simulink model "gm_uz_mpc_cost_and_optim_state_machine"  (R2021a)
settings: Solver=FixedStepAuto  StartTime=0.0  StopTime=10000*t_ADC  RelTol=1e-3
undefined symbols (not defined in the file or in its folder): A, f, IB, id_ref, iq_ref, ix_ref, iy_ref, lambda_d, lambda_q, lambda_u, lambda_x, lambda_y, Ld_over_LB, Lq_over_LB, n_rpm, omega_m, omegaB, p, psi_pm_over_psiB, Rs_over_ZB, t_ADC, t_clock, Ts_times_ZB_over_Ld, Ts_times_ZB_over_Lq, Ts_times_ZB_over_Lx, Ts_times_ZB_over_Ly, v_dc, VB
libraries: hdlmdlgenlib x73, nesl_utility x38, fl_lib x30, ee_lib x14, simulink x10, hdlsllib x2
(part 2 of 3)

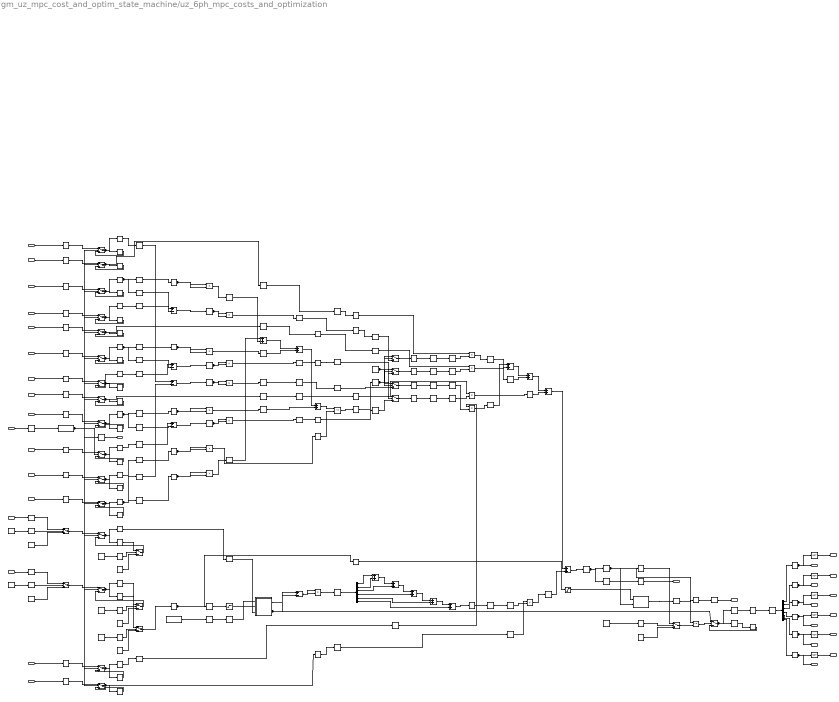
== system gm_uz_mpc_cost_and_optim_state_machine/uz_6ph_mpc_costs_and_optimization ==
  note: squared current error
  note: check for current limit violation
  note: calculate switching effort
  note: calculate costs
  note: find minimum of costs by comparing costs one after another
  note: i_max^2 <= id^2+iq^2+ix^2+iy^2
  id_ref_pu_AXI : Inport  OutDataTypeStr=fixdt(1, 18, 11)  PortDimensions=1  SampleTime=1e-08
  iq_ref_pu_AXI : Inport  Port=2  OutDataTypeStr=fixdt(1, 18, 11)  PortDimensions=1  SampleTime=1e-08
  ix_ref_pu_AXI : Inport  Port=3  OutDataTypeStr=fixdt(1, 18, 11)  PortDimensions=1  SampleTime=1e-08
  iy_ref_pu_AXI : Inport  Port=4  OutDataTypeStr=fixdt(1, 18, 11)  PortDimensions=1  SampleTime=1e-08
  id_pred_pu : Inport  Port=5  OutDataTypeStr=fixdt(1, 27, 16)  PortDimensions=1  SampleTime=1e-08
  iq_pred_pu : Inport  Port=6  OutDataTypeStr=fixdt(1, 27, 16)  PortDimensions=1  SampleTime=1e-08
  ix_pred_pu : Inport  Port=7  OutDataTypeStr=fixdt(1, 18, 11)  PortDimensions=1  SampleTime=1e-08
  iy_pred_pu : Inport  Port=8  OutDataTypeStr=fixdt(1, 18, 11)  PortDimensions=1  SampleTime=1e-08
  max_current_pu_AXI : Inport  Port=9  OutDataTypeStr=fixdt(0, 18, 15)  PortDimensions=1  SampleTime=1e-08
  index : Inport  Port=10  OutDataTypeStr=uint8  PortDimensions=1  SampleTime=1e-08
  last_optim_index : Inport  Port=11  OutDataTypeStr=uint32  PortDimensions=1  SampleTime=1e-08
  lambda_d_AXI : Inport  Port=12  OutDataTypeStr=fixdt(0, 18, 17)  PortDimensions=1  SampleTime=1e-08
  lambda_q_AXI : Inport  Port=13  OutDataTypeStr=fixdt(0, 18, 17)  PortDimensions=1  SampleTime=1e-08
  lambda_x_AXI : Inport  Port=14  OutDataTypeStr=fixdt(0, 18, 17)  PortDimensions=1  SampleTime=1e-08
  lambda_y_AXI : Inport  Port=15  OutDataTypeStr=fixdt(0, 18, 17)  PortDimensions=1  SampleTime=1e-08
  lambda_u_AXI : Inport  Port=16  OutDataTypeStr=fixdt(0, 18, 17)  PortDimensions=1  SampleTime=1e-08
  trigger : Inport  Port=17  OutDataTypeStr=boolean  PortDimensions=1  SampleTime=1e-08
  Add : Sum  Inputs=+-  AccumDataTypeStr=fixdt(1, 28, 16)  OutDataTypeStr=fixdt(1, 28, 16)  SampleTime=1e-08
  Add1 : Sum  Inputs=+-  AccumDataTypeStr=fixdt(1, 28, 16)  OutDataTypeStr=fixdt(1, 28, 16)  SampleTime=1e-08
  Add2 : Sum  Inputs=+-  AccumDataTypeStr=fixdt(1, 19, 11)  OutDataTypeStr=fixdt(1, 19, 11)  SampleTime=1e-08
  Add3 : Sum  Inputs=+-  AccumDataTypeStr=fixdt(1, 19, 11)  OutDataTypeStr=fixdt(1, 19, 11)  SampleTime=1e-08
  Add4_stage2 : Sum  AccumDataTypeStr=fixdt(0, 27, 22)  OutDataTypeStr=fixdt(0, 28, 22)  SampleTime=1e-08
  Add4_stage3 : Sum  AccumDataTypeStr=fixdt(0, 27, 22)  OutDataTypeStr=fixdt(0, 29, 22)  SampleTime=1e-08
  Add4_stage4 : Sum  AccumDataTypeStr=fixdt(0, 27, 22)  OutDataTypeStr=fixdt(0, 27, 22)  SampleTime=1e-08
  Add5 : Sum  Inputs=+-  AccumDataTypeStr=fixdt(1, 9, 0)  OutDataTypeStr=fixdt(1, 9, 0)  SampleTime=1e-08
  Add6_stage2 : Sum  AccumDataTypeStr=fixdt(0, 27, 24)  OutDataTypeStr=fixdt(0, 28, 22)  SampleTime=1e-08
  Add6_stage3 : Sum  AccumDataTypeStr=fixdt(0, 27, 24)  OutDataTypeStr=fixdt(0, 29, 22)  SampleTime=1e-08
  Add6_stage4 : Sum  AccumDataTypeStr=fixdt(0, 27, 24)  OutDataTypeStr=fixdt(0, 30, 22)  SampleTime=1e-08
  Add6_stage5 : Sum  AccumDataTypeStr=fixdt(0, 27, 24)  OutDataTypeStr=fixdt(0, 27, 24)  SampleTime=1e-08
  Delay{,1..23,25..49,51..72,94} (72 alike) : Delay  DelayLength=double(1)  InitialCondition=0  SampleTime=1e-08
  Delay13_Initial_Val : Constant  OutDataTypeStr=uint32  SampleTime=1e-08
  Delay13_ctrl_const : Constant  OutDataTypeStr=boolean  SampleTime=1e-08
  Delay13_ctrl_delay : Delay  DelayLength=double(1)  InitialCondition=0  SampleTime=1e-08
  Delay13_switch : Switch  Criteria=u2 ~= 0  Threshold=double(0)  OutDataTypeStr=uint32  SampleTime=1e-08
  Delay22_Initial_Val : Constant  OutDataTypeStr=uint32  SampleTime=1e-08
  Delay22_ctrl_const : Constant  OutDataTypeStr=boolean  SampleTime=1e-08
  Delay22_ctrl_delay : Delay  DelayLength=double(1)  InitialCondition=0  SampleTime=1e-08
  Delay22_switch : Switch  Criteria=u2 ~= 0  Threshold=double(0)  OutDataTypeStr=uint32  SampleTime=1e-08
  Delay23_Initial_Val : Constant  OutDataTypeStr=uint8  SampleTime=1e-08
  Delay23_ctrl_const : Constant  OutDataTypeStr=boolean  SampleTime=1e-08
  Delay23_ctrl_delay : Delay  DelayLength=double(1)  InitialCondition=0  SampleTime=1e-08
  Delay23_switch : Switch  Criteria=u2 ~= 0  Threshold=double(0)  OutDataTypeStr=uint8  SampleTime=1e-08
  Delay24 : Delay  DelayLength=double(2)  InitialCondition=0  SampleTime=1e-08
  Delay24_Initial_Val : Constant  OutDataTypeStr=uint8  SampleTime=1e-08
  Delay24_ctrl_const : Constant  OutDataTypeStr=boolean  SampleTime=1e-08
  Delay24_ctrl_delay : Delay  DelayLength=double(2)  InitialCondition=0  SampleTime=1e-08
  Delay24_switch : Switch  Criteria=u2 ~= 0  Threshold=double(0)  OutDataTypeStr=uint8  SampleTime=1e-08
  Delay35_Initial_Val : Constant  Value=4.9900000095367431640625  OutDataTypeStr=fixdt(0, 27, 24)  SampleTime=1e-08
  Delay35_ctrl_const : Constant  OutDataTypeStr=boolean  SampleTime=1e-08
  Delay35_ctrl_delay : Delay  DelayLength=double(1)  InitialCondition=0  SampleTime=1e-08
  Delay35_switch : Switch  Criteria=u2 ~= 0  Threshold=double(0)  OutDataTypeStr=fixdt(0, 27, 24)  SampleTime=1e-08
  Delay37_out1_wire : hdlmdlgenlib/Buffer
      settings: SourceProductBaseCode=SL
  Delay38_out1_0_wire : hdlmdlgenlib/Buffer
      settings: SourceProductBaseCode=SL
  Delay38_out1_1_wire : hdlmdlgenlib/Buffer
      settings: SourceProductBaseCode=SL
  Delay38_out1_2_wire : hdlmdlgenlib/Buffer
      settings: SourceProductBaseCode=SL
  Delay38_out1_3_wire : hdlmdlgenlib/Buffer
      settings: SourceProductBaseCode=SL
  Delay38_out1_4_wire : hdlmdlgenlib/Buffer
      settings: SourceProductBaseCode=SL
  Delay38_out1_5_wire : hdlmdlgenlib/Buffer
      settings: SourceProductBaseCode=SL
  Delay50 : Delay  DelayLength=double(4)  InitialCondition=0  SampleTime=1e-08
  Delay50_Initial_Val : Constant  OutDataTypeStr=uint8  SampleTime=1e-08
  Delay50_ctrl_const : Constant  OutDataTypeStr=boolean  SampleTime=1e-08
  Delay50_ctrl_delay : Delay  DelayLength=double(4)  InitialCondition=0  SampleTime=1e-08
  Delay50_switch : Switch  Criteria=u2 ~= 0  Threshold=double(0)  OutDataTypeStr=uint8  SampleTime=1e-08
  Detect Rise Positive : simulink/Logic and Bit Operations/Detect Rise Positive  vinit=0  OutDataTypeStr=boolean
  FiniteControlSetSwitchingTable : Subsystem
  From{,1..34,36} (36 alike) : hdlmdlgenlib/Buffer
      settings: SourceProductBaseCode=SL
  Goto{,1..27,29,47} (30 alike) : hdlmdlgenlib/Buffer
      settings: SourceProductBaseCode=SL
  MATLAB Function : Subsystem
  NOT{,1..5} (6 alike) : Logic  Operator=NOT  Inputs=1  AllPortsSameDT=off  OutDataTypeStr=boolean  SampleTime=1e-08
  Product{,1..7,9..12,14} (13 alike) : Product  Inputs=**  OutDataTypeStr=fixdt(0, 27, 22)  SampleTime=1e-08
  Product13 : Product  Inputs=**  OutDataTypeStr=fixdt(0, 27, 24)  SampleTime=1e-08
  Product8 : Product  Inputs=**  OutDataTypeStr=uint16  SampleTime=1e-08
  Relational Operator : RelationalOperator  OutDataTypeStr=boolean  SampleTime=1e-08  RndMeth=Nearest
  Relational Operator1 : RelationalOperator  Operator=<=  OutDataTypeStr=boolean  SampleTime=1e-08  RndMeth=Nearest
  Saturation : Saturate  UpperLimit="fi(0,0,8,0,\"hex\",\"40\")"  LowerLimit="fi(0,0,8,0,\"hex\",\"01\")"  SampleTime=1e-08  OutDataTypeStr=uint8
  Saturation1 : Saturate  UpperLimit="fi(0,0,8,0,\"hex\",\"40\")"  LowerLimit="fi(0,0,8,0,\"hex\",\"01\")"  SampleTime=1e-08  OutDataTypeStr=uint8
  Sum of Elements_stage2 : Sum  AccumDataTypeStr=uint16  OutDataTypeStr=fixdt(0, 17, 0)  SampleTime=1e-08
  Sum of Elements_stage3 : Sum  AccumDataTypeStr=uint16  OutDataTypeStr=fixdt(0, 18, 0)  SampleTime=1e-08
  Sum of Elements_stage4 : Sum  AccumDataTypeStr=uint16  OutDataTypeStr=fixdt(0, 19, 0)  SampleTime=1e-08
  Sum of Elements_stage5 : Sum  AccumDataTypeStr=uint16  OutDataTypeStr=fixdt(0, 20, 0)  SampleTime=1e-08
  Sum of Elements_stage6 : Sum  AccumDataTypeStr=uint16  OutDataTypeStr=uint16  SampleTime=1e-08
  Switch{,12..14} (4 alike) : Switch  Criteria=u2 > Threshold  Threshold=double(0)  OutDataTypeStr=fixdt(0, 27, 22)  SampleTime=1e-08
  Switch1 : Switch  Criteria=u2 > Threshold  Threshold=double(0)  OutDataTypeStr=fixdt(1, 27, 16)  SampleTime=1e-08
  Switch10 : Switch  Criteria=u2 > Threshold  Threshold=double(0)  OutDataTypeStr=uint32  SampleTime=1e-08
  Switch11 : Switch  Criteria=u2 > Threshold  Threshold=double(0)  OutDataTypeStr=uint8  SampleTime=1e-08
  Switch{15..19} (5 alike) : Switch  Criteria=u2 > Threshold  Threshold=double(0)  OutDataTypeStr=fixdt(0, 18, 17)  SampleTime=1e-08
  Switch2 : Switch  Criteria=u2 > Threshold  Threshold=double(0)  OutDataTypeStr=fixdt(1, 27, 16)  SampleTime=1e-08
  Switch21 : Switch  Criteria=u2 > Threshold  Threshold=double(0)  OutDataTypeStr=boolean  SampleTime=1e-08
  Switch{3..4,6..9} (6 alike) : Switch  Criteria=u2 > Threshold  Threshold=double(0)  OutDataTypeStr=fixdt(1, 18, 11)  SampleTime=1e-08
  Switch5 : Switch  Criteria=u2 > Threshold  Threshold=double(0)  OutDataTypeStr=fixdt(0, 18, 15)  SampleTime=1e-08
  iterativesearch : Subsystem
  sfix18_En15 max value : Constant  Value=3.989990234375  OutDataTypeStr=fixdt(1, 18, 15)  SampleTime=1e-08
  t : Demux  Outputs=6
  t1 : Demux  Outputs=6
  opt_index : Outport  SampleTime=1e-08  VectorParamsAs1DForOutWhenUnconnected=off
  G0 : Outport  Port=2  SampleTime=1e-08  VectorParamsAs1DForOutWhenUnconnected=off
  G1 : Outport  Port=3  SampleTime=1e-08  VectorParamsAs1DForOutWhenUnconnected=off
  G2 : Outport  Port=4  SampleTime=1e-08  VectorParamsAs1DForOutWhenUnconnected=off
  G3 : Outport  Port=5  SampleTime=1e-08  VectorParamsAs1DForOutWhenUnconnected=off
  G4 : Outport  Port=6  SampleTime=1e-08  VectorParamsAs1DForOutWhenUnconnected=off
  G5 : Outport  Port=7  SampleTime=1e-08  VectorParamsAs1DForOutWhenUnconnected=off
  G6 : Outport  Port=8  SampleTime=1e-08  VectorParamsAs1DForOutWhenUnconnected=off
  G7 : Outport  Port=9  SampleTime=1e-08  VectorParamsAs1DForOutWhenUnconnected=off
  G8 : Outport  Port=10  SampleTime=1e-08  VectorParamsAs1DForOutWhenUnconnected=off
  G9 : Outport  Port=11  SampleTime=1e-08  VectorParamsAs1DForOutWhenUnconnected=off
  G10 : Outport  Port=12  SampleTime=1e-08  VectorParamsAs1DForOutWhenUnconnected=off
  G11 : Outport  Port=13  SampleTime=1e-08  VectorParamsAs1DForOutWhenUnconnected=off
  opt_done : Outport  Port=14  SampleTime=1e-08  VectorParamsAs1DForOutWhenUnconnected=off
  costs : Outport  Port=15  SampleTime=1e-08  VectorParamsAs1DForOutWhenUnconnected=off
  wires:
  id_ref_pu_AXI/1 -> Delay14/1
  iq_ref_pu_AXI/1 -> Delay16/1
  ix_ref_pu_AXI/1 -> Delay18/1
  iy_ref_pu_AXI/1 -> Delay20/1
  id_pred_pu/1 -> Delay2/1
  iq_pred_pu/1 -> Delay5/1
  ix_pred_pu/1 -> Delay7/1
  iy_pred_pu/1 -> Delay9/1
  max_current_pu_AXI/1 -> Delay12/1
  index/1 -> Delay24/1
  last_optim_index/1 -> Delay22/1
  lambda_d_AXI/1 -> Delay26/1
  lambda_q_AXI/1 -> Delay28/1
  lambda_x_AXI/1 -> Delay30/1
  lambda_y_AXI/1 -> Delay32/1
  lambda_u_AXI/1 -> Delay34/1
  trigger/1 -> Delay/1
  Add/1 -> Delay46/1
  Add1/1 -> Delay47/1
  Add2/1 -> Delay48/1
  Add3/1 -> Delay49/1
  Add4_stage4/1 -> Relational Operator/1
  Add5/1 -> Product8/2, Product8/1
  Add6_stage5/1 -> Goto27/1
  Delay/1 -> Detect Rise Positive/1
  Delay1/1 -> opt_done/1
  Delay10/1 -> Switch4/3
  Delay11/1 -> Switch5/3
  Delay12/1 -> Switch5/1
  Delay13_switch/1 -> Switch10/3
  Delay14/1 -> Switch6/1
  Delay15/1 -> Switch6/3
  Delay16/1 -> Switch7/1
  Delay17/1 -> Switch7/3
  Delay18/1 -> Switch8/1
  Delay19/1 -> Switch8/3
  Delay2/1 -> Switch1/1
  Delay20/1 -> Switch9/1
  Delay21/1 -> Switch9/3
  Delay22_switch/1 -> Switch10/1
  Delay23_switch/1 -> Switch11/3
  Delay24_switch/1 -> Switch11/1
  Delay25/1 -> Switch15/3
  Delay26/1 -> Switch15/1
  Delay27/1 -> Switch16/3
  Delay28/1 -> Switch16/1
  Delay29/1 -> Switch17/3
  Delay3/1 -> Switch1/3
  Delay30/1 -> Switch17/1
  Delay31/1 -> Switch18/3
  Delay32/1 -> Switch18/1
  Delay33/1 -> Switch19/3
  Delay34/1 -> Switch19/1
  Delay35_switch/1 -> Relational Operator1/2
  Delay36/1 -> Product4/2, Product4/1
  Delay37/1 -> Delay37_out1_wire/1
  Delay38/1 -> t/1
  Delay39/1 -> Product5/2, Product5/1
  Delay4/1 -> opt_index/1
  Delay40/1 -> Product6/2, Product6/1
  Delay41/1 -> Product7/2, Product7/1
  Delay42/1 -> Add4_stage2/1
  Delay43/1 -> Add4_stage2/2
  Delay44/1 -> Add4_stage3/2
  Delay45/1 -> Add4_stage4/2
  Delay46/1 -> Product/2, Product/1
  Delay47/1 -> Product1/2, Product1/1
  Delay48/1 -> Product2/2, Product2/1
  Delay49/1 -> Product3/2, Product3/1
  Delay5/1 -> Switch2/1
  Delay50_switch/1 -> Goto2/1
  Delay51/1 -> Product14/2, Product14/1
  Delay52/1 -> Relational Operator/2
  Delay53/1 -> Add6_stage2/1
  Delay54/1 -> Add6_stage2/2
  Delay55/1 -> Add6_stage3/2
  Delay56/1 -> Add6_stage4/2
  Delay57/1 -> Add6_stage5/2
  Delay58/1 -> t1/1
  Delay59/1 -> Product9/2
  Delay6/1 -> Switch2/3
  Delay60/1 -> Product10/2
  Delay61/1 -> Product11/2
  Delay62/1 -> Product12/2
  Delay63/1 -> Product13/2
  Delay64/1 -> Product9/1
  Delay65/1 -> Product10/1
  Delay66/1 -> Product11/1
  Delay67/1 -> Product12/1
  Delay68/1 -> Product13/1
  Delay69/1 -> Goto10/1
  Delay7/1 -> Switch3/1
  Delay70/1 -> Goto11/1
  Delay71/1 -> Goto12/1
  Delay72/1 -> Goto13/1
  Delay8/1 -> Switch3/3
  Delay9/1 -> Switch4/1
  Delay94/1 -> costs/1
  Delay38_out1_0_wire/1 -> NOT/1, G0/1
  Delay38_out1_1_wire/1 -> NOT1/1, G2/1
  Delay38_out1_2_wire/1 -> NOT2/1, G4/1
  Delay38_out1_3_wire/1 -> NOT3/1, G6/1
  Delay38_out1_4_wire/1 -> NOT4/1, G8/1
  Delay38_out1_5_wire/1 -> NOT5/1, G10/1
  Detect Rise Positive/1 -> Switch9/2, Switch8/2, Switch7/2, Switch6/2, Switch5/2, Switch4/2, Switch3/2, Switch2/2, Switch19/2, Switch18/2, Switch17/2, Switch16/2, Switch15/2, Switch11/2, Switch10/2, Switch1/2, Delay1/1
  FiniteControlSetSwitchingTable/1(G) -> Goto47/1
  From/1 -> Add/1
  From1/1 -> Add/2
  From10/1 -> Switch/3
  From11/1 -> Switch14/2, Switch13/2, Switch12/2, Switch/2
  From12/1 -> Switch12/3
  From13/1 -> Switch13/3
  From14/1 -> Delay36/1
  From15/1 -> Delay39/1
  From16/1 -> Delay40/1
  From17/1 -> Delay41/1
  From18/1 -> Switch14/3
  From19/1 -> Saturation/1
  From2/1 -> Delay94/1
  From20/1 -> MATLAB Function/1(in)
  From21/1 -> MATLAB Function/3(last_optim_index)
  From22/1 -> Delay59/1
  From23/1 -> Delay60/1
  From24/1 -> Delay61/1
  From25/1 -> Delay62/1
  From26/1 -> Delay64/1
  From27/1 -> Delay65/1
  From28/1 -> Delay66/1
  From29/1 -> Delay67/1
  From3/1 -> Add1/2
  From30/1 -> Delay68/1
  From31/1 -> Delay63/1
  From32/1 -> Saturation1/1
  From33/1 -> Relational Operator1/1, Delay35/1, iterativesearch/2(cost)
  From34/1 -> Delay4/1
  From36/1 -> Delay38/1
  From4/1 -> Add2/2
  From5/1 -> Add3/2
  From6/1 -> Add3/1
  From7/1 -> Add2/1
  From8/1 -> Add1/1
  From9/1 -> Delay51/1
  MATLAB Function/1(G_next) -> Add5/2
  MATLAB Function/2(G_prev) -> Switch21/1, Add5/1
  NOT/1 -> G1/1
  NOT1/1 -> G3/1
  NOT2/1 -> G5/1
  NOT3/1 -> G7/1
  NOT4/1 -> G9/1
  NOT5/1 -> G11/1
  Product/1 -> Delay69/1
  Product1/1 -> Delay70/1
  Product10/1 -> Delay54/1
  Product11/1 -> Delay55/1
  Product12/1 -> Delay56/1
  Product13/1 -> Delay57/1
  Product14/1 -> Delay52/1
  Product2/1 -> Delay71/1
  Product3/1 -> Delay72/1
  Product4/1 -> Delay42/1
  Product5/1 -> Delay43/1
  Product6/1 -> Delay44/1
  Product7/1 -> Delay45/1
  Product8/1 -> Delay58/1
  Product9/1 -> Delay53/1
  Relational Operator/1 -> Goto14/1
  Relational Operator1/1 -> Switch21/2
  Saturation/1 -> MATLAB Function/2(index)
  Saturation1/1 -> iterativesearch/1(index)
  Sum of Elements_stage6/1 -> Goto21/1
  Switch/1 -> Goto15/1
  Switch1/1 -> Goto1/1, Delay3/1
  Switch10/1 -> Goto20/1, Delay13/1
  Switch11/1 -> Delay50/1, Delay23/1
  Switch12/1 -> Goto16/1
  Switch13/1 -> Goto17/1
  Switch14/1 -> Goto18/1
  Switch15/1 -> Goto22/1, Delay25/1
  Switch16/1 -> Goto23/1, Delay27/1
  Switch17/1 -> Goto24/1, Delay29/1
  Switch18/1 -> Goto25/1, Delay31/1
  Switch19/1 -> Goto26/1, Delay33/1
  Switch2/1 -> Goto6/1, Delay6/1
  Switch21/1 -> Goto29/1, Delay37/1
  Switch3/1 -> Goto7/1, Delay8/1
  Switch4/1 -> Goto8/1, Delay10/1
  Switch5/1 -> Goto9/1, Delay11/1
  Switch6/1 -> Goto/1, Delay15/1
  Switch7/1 -> Goto3/1, Delay17/1
  Switch8/1 -> Goto4/1, Delay19/1
  Switch9/1 -> Goto5/1, Delay21/1
  iterativesearch/1(opt_idx) -> Goto19/1
  sfix18_En15 max value/1 -> Switch14/1, Switch13/1, Switch12/1, Switch/1
  Goto/1 -> From/1
  Goto1/1 -> From14/1, From1/1
  Goto10/1 -> From10/1
  Goto14/1 -> From11/1
  Goto11/1 -> From12/1
  Goto12/1 -> From13/1
  Goto6/1 -> From3/1, From15/1
  Goto7/1 -> From4/1, From16/1
  Goto8/1 -> From5/1, From17/1
  Goto13/1 -> From18/1
  Goto2/1 -> From32/1, From19/1
  Goto27/1 -> From33/1, From2/1
  Goto47/1 -> From20/1
  Goto20/1 -> From21/1
  Goto15/1 -> From22/1
  Goto16/1 -> From23/1
  Goto17/1 -> From24/1
  Goto18/1 -> From25/1
  Goto22/1 -> From26/1
  Goto23/1 -> From27/1
  Goto24/1 -> From28/1
  Goto25/1 -> From29/1
  Goto26/1 -> From30/1
  Goto21/1 -> From31/1
  Goto19/1 -> From34/1
  Goto29/1 -> From36/1
  Goto5/1 -> From6/1
  Goto4/1 -> From7/1
  Goto3/1 -> From8/1
  Goto9/1 -> From9/1
  Delay13/1 -> Delay13_switch/1
  Delay13_Initial_Val/1 -> Delay13_switch/3
  Delay13_ctrl_const/1 -> Delay13_ctrl_delay/1
  Delay13_ctrl_delay/1 -> Delay13_switch/2
  Delay22/1 -> Delay22_switch/1
  Delay22_Initial_Val/1 -> Delay22_switch/3
  Delay22_ctrl_const/1 -> Delay22_ctrl_delay/1
  Delay22_ctrl_delay/1 -> Delay22_switch/2
  Delay23/1 -> Delay23_switch/1
  Delay23_Initial_Val/1 -> Delay23_switch/3
  Delay23_ctrl_const/1 -> Delay23_ctrl_delay/1
  Delay23_ctrl_delay/1 -> Delay23_switch/2
  Delay24/1 -> Delay24_switch/1
  Delay24_Initial_Val/1 -> Delay24_switch/3
  Delay24_ctrl_const/1 -> Delay24_ctrl_delay/1
  Delay24_ctrl_delay/1 -> Delay24_switch/2
  Delay35/1 -> Delay35_switch/1
  Delay35_Initial_Val/1 -> Delay35_switch/3
  Delay35_ctrl_const/1 -> Delay35_ctrl_delay/1
  Delay35_ctrl_delay/1 -> Delay35_switch/2
  Delay50/1 -> Delay50_switch/1
  Delay50_Initial_Val/1 -> Delay50_switch/3
  Delay50_ctrl_const/1 -> Delay50_ctrl_delay/1
  Delay50_ctrl_delay/1 -> Delay50_switch/2
  Add4_stage2/1 -> Add4_stage3/1
  Add4_stage3/1 -> Add4_stage4/1
  Add6_stage2/1 -> Add6_stage3/1
  Add6_stage3/1 -> Add6_stage4/1
  Add6_stage4/1 -> Add6_stage5/1
  t/1 -> Delay38_out1_0_wire/1
  t/2 -> Delay38_out1_1_wire/1
  t/3 -> Delay38_out1_2_wire/1
  t/4 -> Delay38_out1_3_wire/1
  t/5 -> Delay38_out1_4_wire/1
  t/6 -> Delay38_out1_5_wire/1
  t1/1 -> Sum of Elements_stage2/1
  t1/2 -> Sum of Elements_stage2/2
  t1/3 -> Sum of Elements_stage3/2
  t1/4 -> Sum of Elements_stage4/2
  t1/5 -> Sum of Elements_stage5/2
  t1/6 -> Sum of Elements_stage6/2
  Sum of Elements_stage2/1 -> Sum of Elements_stage3/1
  Sum of Elements_stage3/1 -> Sum of Elements_stage4/1
  Sum of Elements_stage4/1 -> Sum of Elements_stage5/1
  Sum of Elements_stage5/1 -> Sum of Elements_stage6/1
  Delay37_out1_wire/1 -> Switch21/3

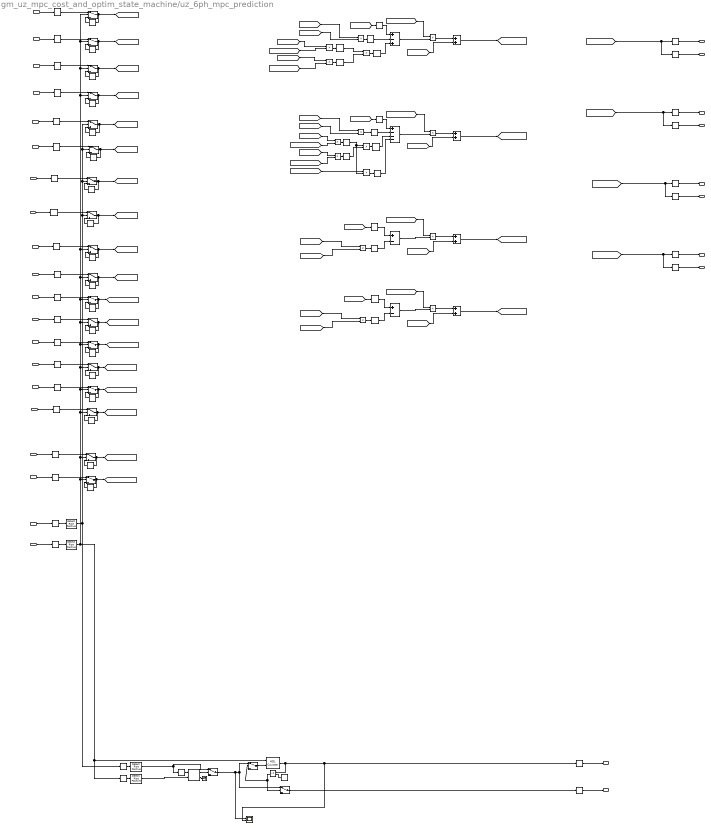
== system gm_uz_mpc_cost_and_optim_state_machine/uz_6ph_mpc_prediction ==
  note: mpc state machine
  note: id_delay_pu = Ts_times_ZB_over_Ld *(vd_pu - Rs_over_ZB * id_k_pu + iq_k_pu * Lq_over_LB * omega_m_pu * polepairs) + id_k_pu
  note: iq_delay_pu = Ts_times_ZB_over_Lq *(vq_pu - Rs_over_ZB * iq_k_pu - omega_m_pu * polepairs * Ld_over_LB * id_k_pu - omega_m_pu * polepairs * psi_pm_over_psiB) + iq_k_pu
  note: ix_delay_pu = Ts_times_ZB_over_Lx *(vx_pu - Rs_over_ZB* ix_k_pu) + ix_k_pu
  note: iy_delay_pu = Ts_times_ZB_over_Ly *(vy_pu - Rs_over_ZB * iy_k_pu) + iy_k_pu
  note: voltages are triggered from voltage calculation ip every iteration
  id_pu : Inport  OutDataTypeStr=fixdt_type_dq_currents
  iq_pu : Inport  Port=2  OutDataTypeStr=fixdt_type_dq_currents
  ix_pu : Inport  Port=3  OutDataTypeStr=fixdt_type_xy_currents
  iy_pu : Inport  Port=4  OutDataTypeStr=fixdt_type_xy_currents
  vd_pu : Inport  Port=5  OutDataTypeStr=fixdt_type_dqxy_voltages
  vq_pu : Inport  Port=6  OutDataTypeStr=fixdt_type_dqxy_voltages
  vx_pu : Inport  Port=7  OutDataTypeStr=fixdt_type_dqxy_voltages
  vy_pu : Inport  Port=8  OutDataTypeStr=fixdt_type_dqxy_voltages
  omega_m_pu : Inport  Port=9  OutDataTypeStr=fixdt_type_speed
  Rs_over_ZB_AXI : Inport  Port=10  OutDataTypeStr=fixdt_type_constants
  Ts_times_ZB_over_Ld_AXI : Inport  Port=11  OutDataTypeStr=fixdt_type_constants
  Ts_times_ZB_over_Lq_AXI : Inport  Port=12  OutDataTypeStr=fixdt_type_constants
  Ts_times_ZB_over_Lx_AXI : Inport  Port=13  OutDataTypeStr=fixdt_type_constants
  Ts_times_ZB_over_Ly_AXI : Inport  Port=14  OutDataTypeStr=fixdt_type_constants
  Ld_over_LB_AXI : Inport  Port=15  OutDataTypeStr=fixdt_type_constants
  Lq_over_LB_AXI : Inport  Port=16  OutDataTypeStr=fixdt_type_constants
  psi_pm_over_psiB_AXI : Inport  Port=17  OutDataTypeStr=fixdt_type_constants
  polepairs_AXI : Inport  Port=18  OutDataTypeStr=fixdt_type_polepairs
  trigger_voltages_done : Inport  Port=19
  adc_trigger : Inport  Port=20
  Add : Sum  Inputs=+-+  AccumDataTypeStr=fixdt(1,27,16)
  Add{1,3,5,7} (4 alike) : Sum  AccumDataTypeStr=fixdt(1,27,24)
  Add2 : Sum  Inputs=+---  AccumDataTypeStr=fixdt(1,27,16)
  Add4 : Sum  Inputs=+-  AccumDataTypeStr=fixdt(1,27,16)
  Add6 : Sum  Inputs=+-  AccumDataTypeStr=fixdt(1,27,16)
  Constant : Constant  Value=63  OutDataTypeStr=uint8  SampleTime=-1
  Delay{,2,4,6,8,11..12,14..17,25,27,29,31,33,35,37,39,43,50,59..60,62..65,71,73} (29 alike) : Delay
  Delay{1,3,5,7,9..10,13,18..24,26,28,30,32,34,36,38,40..42,44..48,53..55,57..58,70,72} (36 alike) : Delay  DelayLength=1
  Delay49 : Delay  DelayLength=1  InitialCondition=0
  Detect Rise Positive{,1..3} (4 alike) : simulink/Logic and Bit Operations/Detect Rise Positive  vinit=0  OutDataTypeStr=boolean
  HDL Counter : hdlsllib/Sources/HDL Counter  CountType=Free running  CountInit=0  CountStep=1  CountMax=64  CountFromType=Initial value  CountFrom=0  CountResetPort=on  CountLoadPort=off  CountEnbPort=on  CountDirPort=off  CountHitOutputPort=off  CountDataType=Unsigned  CountWordLen=8  CountFracLen=0  CountSampTime=1
  Product{,1..2,4..7,9..14} (13 alike) : Product  OutDataTypeStr=fixdt(1,18,15)
  Product3 : Product  OutDataTypeStr=fixdt(1,27,16)
  Product8 : Product  OutDataTypeStr=fixdt(1,27,16)
  Relational Operator : RelationalOperator  Operator=<=  OutDataTypeStr=boolean  RndMeth=Simplest
  Scope : Scope  NumInputPorts=2
  Subsystem : Subsystem
  Switch : Switch  Criteria=u2 > Threshold  OutDataTypeStr=fixdt_type_dq_currents
  Switch1 : Switch  Criteria=u2 > Threshold  OutDataTypeStr=fixdt_type_dq_currents
  Switch{12..19} (8 alike) : Switch  Criteria=u2 > Threshold  OutDataTypeStr=fixdt_type_constants
  Switch2 : Switch  Criteria=u2 > Threshold  OutDataTypeStr=fixdt_type_xy_currents
  Switch21 : Switch  Criteria=u2 > Threshold  OutDataTypeStr=fixdt_type_polepairs
  Switch{28..31} (4 alike) : Switch  Criteria=u2 > Threshold  OutDataTypeStr=fixdt_type_dqxy_voltages
  Switch3 : Switch  Criteria=u2 > Threshold  OutDataTypeStr=fixdt_type_xy_currents
  Switch4 : Switch  Criteria=u2 > Threshold
  Switch5 : Switch  Criteria=u2 > Threshold  OutDataTypeStr=fixdt_type_speed
  Switch6 : Switch  Criteria=u2 > Threshold
  Switch7 : Switch  Criteria=u2 > Threshold
  Terminator1 : Terminator
  id_pred_pu : Outport
  iq_pred_pu : Outport  Port=2
  ix_pred_pu : Outport  Port=3
  iy_pred_pu : Outport  Port=4
  id_pred_pu_AXI : Outport  Port=5
  iq_pred_pu_AXI : Outport  Port=6
  ix_pred_pu_AXI : Outport  Port=7
  iy_pred_pu_AXI : Outport  Port=8
  prediction_done : Outport  Port=9
  index : Outport  Port=10  VectorParamsAs1DForOutWhenUnconnected=off
  wires:
  Switch6/1 -> Delay11/1
  Relational Operator/1 -> Switch4/2, Switch6/2
  Switch4/1 -> HDL Counter/2
  Constant/1 -> Relational Operator/2
  Delay49/1 -> index/1
  HDL Counter/1 -> Delay49/1, Scope/2, Relational Operator/1
  Delay53/1 -> Detect Rise Positive2/1
  Subsystem/1(Q) -> Switch7/2  "Q"
  Detect Rise Positive2/1 -> Switch7/1, Delay55/1
  Subsystem/2(!Q) -> Terminator1/1
  Delay55/1 -> Subsystem/1(Set)
  Delay54/1 -> Detect Rise Positive3/1
  Detect Rise Positive3/1 -> Subsystem/2(Reset)
  Detect Rise Positive/1 -> HDL Counter/1, Delay54/1, Switch/2, Switch1/2, Switch2/2, Switch3/2, Switch5/2, Switch12/2, Switch13/2, Switch14/2, Switch15/2, Switch16/2, Switch17/2, Switch18/2, Switch19/2, Switch21/2
  Switch7/1 -> Switch4/1, Switch6/1, Scope/1  "trigger_predict"
  Delay50/1 -> Detect Rise Positive1/1
  trigger_voltages_done/1 -> Delay50/1
  Detect Rise Positive1/1 -> Switch28/2, Switch29/2, Switch30/2, Switch31/2, Delay53/1  "delay_comp done"
  Delay48/1 -> Product7/2
  Product8/1 -> Delay48/1
  Delay47/1 -> Product7/1, Product10/2
  Product9/1 -> Delay47/1
  Delay45/1 -> Product2/1
  Delay46/1 -> Product2/2
  Product3/1 -> Delay46/1
  Product4/1 -> Delay45/1
  Delay41/1 -> Add6/1
  Delay42/1 -> Add6/2
  Product14/1 -> Delay42/1
  [vy_pu] -> Delay41/1  "vy_pu"
  Delay24/1 -> Add4/2
  Product12/1 -> Delay24/1
  Delay23/1 -> Add4/1
  [vx_pu] -> Delay23/1  "vx_pu"
  Product6/1 -> Delay20/1
  Delay19/1 -> Add2/1
  Delay20/1 -> Add2/2
  Delay21/1 -> Add2/3
  Delay22/1 -> Add2/4
  Product10/1 -> Delay22/1
  Product7/1 -> Delay21/1
  [vq_pu] -> Delay19/1  "vq_pu"
  Delay18/1 -> Add/1
  [vd_pu] -> Delay18/1  "vd_pu"
  Delay1/1 -> Add/3
  Delay10/1 -> Add/2
  Product1/1 -> Delay10/1
  Product2/1 -> Delay1/1
  Product13/1 -> Add7/1
  [Ts_times_ZB_over_Ly_AXI] -> Product13/1  "Ts_times_ZB_over_Ly"
  [iy_pu] -> Product14/2  "iy_k_pu"
  [iy_pu] -> Add7/2  "iy_k_pu"
  Add6/1 -> Product13/2
  [Rs_over_ZB_AXI] -> Product14/1  "Rs_over_ZB"
  Product11/1 -> Add5/1
  [ix_pu] -> Add5/2  "ix_k_pu"
  Add4/1 -> Product11/2
  [Rs_over_ZB_AXI] -> Product12/1  "Rs_over_ZB"
  [ix_pu] -> Product12/2  "ix_k_pu"
  [Ts_times_ZB_over_Lx_AXI] -> Product11/1  "Ts_times_ZB_over_Lx"
  [psi_pm_over_psiB_AXI] -> Product10/1
  Product5/1 -> Add3/1
  [polepairs_AXI] -> Product9/2  "polepairs"
  [Ld_over_LB_AXI] -> Product8/2  "Ld_over_LB"
  [id_pu] -> Product8/1  "id_k_pu"
  [iq_pu] -> Add3/2  "iq_k_pu"
  [omega_m_pu] -> Product9/1  "omega_m_pu"
  Add2/1 -> Product5/2
  [Rs_over_ZB_AXI] -> Product6/1  "Rs_over_ZB"
  [iq_pu] -> Product6/2  "iq_k_pu"
  [Ts_times_ZB_over_Lq_AXI] -> Product5/1  "Ts_times_ZB_over_Lq"
  [polepairs_AXI] -> Product4/2  "polepairs"
  [omega_m_pu] -> Product4/1  "omega_m_pu"
  [Lq_over_LB_AXI] -> Product3/2  "Lq_over_LB"
  [iq_pu] -> Product3/1  "iq_k_pu"
  [id_pu] -> Product1/2  "id_k_pu"
  [Rs_over_ZB_AXI] -> Product1/1  "Rs_over_ZB"
  [id_pu] -> Add1/2  "id_k_pu"
  Product/1 -> Add1/1
  [Ts_times_ZB_over_Ld_AXI] -> Product/1  "Ts_times_ZB_over_Ld"
  Add/1 -> Product/2
  Delay17/1 -> iy_pred_pu/1
  Delay16/1 -> ix_pred_pu/1
  Delay14/1 -> id_pred_pu/1
  Delay15/1 -> iq_pred_pu/1
  Delay62/1 -> id_pred_pu_AXI/1
  [ix_delay_pu] -> Delay64/1, Delay16/1
  Delay64/1 -> ix_pred_pu_AXI/1
  Delay65/1 -> iy_pred_pu_AXI/1
  Delay63/1 -> iq_pred_pu_AXI/1
  [id_delay_pu] -> Delay62/1, Delay14/1
  [iq_delay_pu] -> Delay63/1, Delay15/1
  [iy_delay_pu] -> Delay65/1, Delay17/1
  Delay11/1 -> prediction_done/1
  Delay30/1 -> Switch14/3
  Delay36/1 -> Switch17/3
  Delay32/1 -> Switch15/3
  Delay13/1 -> Switch5/3
  Delay40/1 -> Switch19/3
  adc_trigger/1 -> Delay/1
  Delay39/1 -> Switch19/1
  Rs_over_ZB_AXI/1 -> Delay25/1
  Delay57/1 -> Switch28/3
  Ts_times_ZB_over_Ld_AXI/1 -> Delay27/1
  Switch1/1 -> Delay5/1, [iq_pu]
  Delay71/1 -> Switch30/1
  Ts_times_ZB_over_Lx_AXI/1 -> Delay31/1
  Switch19/1 -> Delay40/1, [psi_pm_over_psiB_AXI]
  Delay26/1 -> Switch12/3
  Switch18/1 -> [Lq_over_LB_AXI], Delay38/1
  Delay3/1 -> Switch/3
  Ts_times_ZB_over_Lq_AXI/1 -> Delay29/1
  Switch30/1 -> [vx_pu], Delay70/1
  Delay60/1 -> Switch29/1
  Delay70/1 -> Switch30/3
  vy_pu/1 -> Delay73/1
  iy_pu/1 -> Delay8/1
  iq_pu/1 -> Delay4/1
  Lq_over_LB_AXI/1 -> Delay37/1
  Switch5/1 -> Delay13/1, [omega_m_pu]
  vq_pu/1 -> Delay60/1
  Delay27/1 -> Switch13/1
  Delay6/1 -> Switch2/1
  omega_m_pu/1 -> Delay12/1
  Switch31/1 -> [vy_pu], Delay72/1
  Delay73/1 -> Switch31/1
  Delay12/1 -> Switch5/1
  Switch2/1 -> Delay7/1, [ix_pu]
  Delay4/1 -> Switch1/1
  Delay37/1 -> Switch18/1
  Delay7/1 -> Switch2/3
  Ts_times_ZB_over_Ly_AXI/1 -> Delay33/1
  Switch28/1 -> Delay57/1, [vd_pu]
  Delay31/1 -> Switch15/1
  Delay35/1 -> Switch17/1
  Switch/1 -> Delay3/1, [id_pu]
  Switch21/1 -> Delay44/1, [polepairs_AXI]
  id_pu/1 -> Delay2/1
  Delay58/1 -> Switch29/3
  psi_pm_over_psiB_AXI/1 -> Delay39/1
  Delay28/1 -> Switch13/3
  Switch14/1 -> Delay30/1, [Ts_times_ZB_over_Lq_AXI]
  Delay43/1 -> Switch21/1
  Delay72/1 -> Switch31/3
  polepairs_AXI/1 -> Delay43/1
  Switch3/1 -> Delay9/1, [iy_pu]
  Switch29/1 -> Delay58/1, [vq_pu]
  Delay8/1 -> Switch3/1
  Delay29/1 -> Switch14/1
  Delay44/1 -> Switch21/3
  Delay34/1 -> Switch16/3
  Delay/1 -> Detect Rise Positive/1
  Switch13/1 -> Delay28/1, [Ts_times_ZB_over_Ld_AXI]
  Delay9/1 -> Switch3/3
  Switch17/1 -> [Ld_over_LB_AXI], Delay36/1
  Delay38/1 -> Switch18/3
  ix_pu/1 -> Delay6/1
  Switch16/1 -> [Ts_times_ZB_over_Ly_AXI], Delay34/1
  Delay2/1 -> Switch/1
  Ld_over_LB_AXI/1 -> Delay35/1
  Switch15/1 -> Delay32/1, [Ts_times_ZB_over_Lx_AXI]
  vd_pu/1 -> Delay59/1
  vx_pu/1 -> Delay71/1
  Delay33/1 -> Switch16/1
  Delay59/1 -> Switch28/1
  Delay25/1 -> Switch12/1
  Delay5/1 -> Switch1/3
  Add7/1 -> [iy_delay_pu]
  Add1/1 -> [id_delay_pu]
  Add3/1 -> [iq_delay_pu]
  Switch12/1 -> Delay26/1, [Rs_over_ZB_AXI]
  Add5/1 -> [ix_delay_pu]

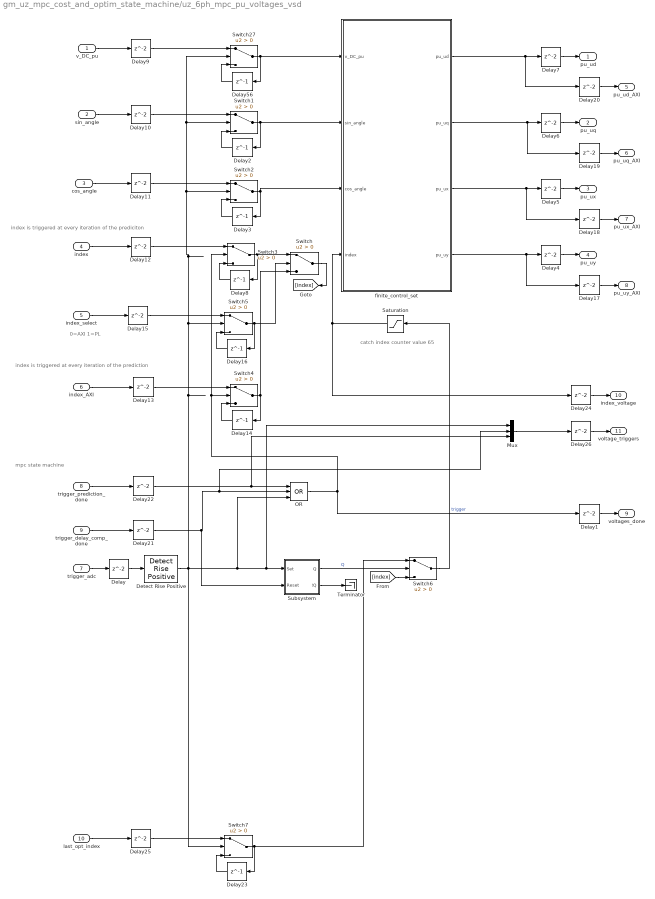
== system gm_uz_mpc_cost_and_optim_state_machine/uz_6ph_mpc_pu_voltages_vsd ==
  note: mpc state machine
  note: 0=AXI 1=PL
  note: index is triggered at every iteration of the prediciton
  note: index is triggered at every iteration of the prediction
  note: catch index counter value 65
  v_DC_pu : Inport  OutDataTypeStr=fixdt_type_constants
  sin_angle : Inport  Port=2  OutDataTypeStr=fixdt_type_sin_cos
  cos_angle : Inport  Port=3  OutDataTypeStr=fixdt_type_sin_cos
  index : Inport  Port=4
  index_select : Inport  Port=5
  index_AXI : Inport  Port=6
  trigger_adc : Inport  Port=7
  trigger_prediction_done : Inport  Port=8
  trigger_delay_comp_done : Inport  Port=9
  last_opt_index : Inport  Port=10
  Delay{,1,4..7,9..11,17..22,24..26} (18 alike) : Delay
  Delay12 : Delay  InitialCondition=0
  Delay13 : Delay  InitialCondition=0
  Delay14 : Delay  DelayLength=1  InitialCondition=0
  Delay15 : Delay  InitialCondition=1
  Delay16 : Delay  DelayLength=1  InitialCondition=1
  Delay2 : Delay  DelayLength=1
  Delay23 : Delay  DelayLength=1  InitialCondition=1
  Delay3 : Delay  DelayLength=1
  Delay56 : Delay  DelayLength=1
  Delay8 : Delay  DelayLength=1  InitialCondition=0
  Detect Rise Positive : simulink/Logic and Bit Operations/Detect Rise Positive  vinit=0  OutDataTypeStr=boolean
  Mux : Mux  Inputs=3
  OR : Logic  Operator=OR  Inputs=3  IconShape=distinctive  AllPortsSameDT=off  OutDataTypeStr=boolean
  Saturation : Saturate  UpperLimit=64  LowerLimit=1
  Subsystem : Subsystem
  Switch : Switch  Criteria=u2 > Threshold
  Switch1 : Switch  Criteria=u2 > Threshold  OutDataTypeStr=fixdt_type_sin_cos
  Switch2 : Switch  Criteria=u2 > Threshold  OutDataTypeStr=fixdt_type_sin_cos
  Switch27 : Switch  Criteria=u2 > Threshold  OutDataTypeStr=fixdt_type_constants
  Switch3 : Switch  Criteria=u2 > Threshold  OutDataTypeStr=fixdt_type_polepairs
  Switch4 : Switch  Criteria=u2 > Threshold  OutDataTypeStr=fixdt_type_polepairs
  Switch5 : Switch  Criteria=u2 > Threshold  OutDataTypeStr=fixdt_type_polepairs
  Switch6 : Switch  Criteria=u2 > Threshold
  Switch7 : Switch  Criteria=u2 > Threshold  OutDataTypeStr=uint32
  Terminator : Terminator
  finite_control_set : MATLAB Function  TreatAsAtomicUnit=on
  pu_ud : Outport
  pu_uq : Outport  Port=2
  pu_ux : Outport  Port=3
  pu_uy : Outport  Port=4
  pu_ud_AXI : Outport  Port=5
  pu_uq_AXI : Outport  Port=6
  pu_ux_AXI : Outport  Port=7
  pu_uy_AXI : Outport  Port=8
  voltages_done : Outport  Port=9
  index_voltage : Outport  Port=10
  voltage_triggers : Outport  Port=11
  wires:
  Mux/1 -> Delay26/1
  Delay26/1 -> voltage_triggers/1
  Delay22/1 -> OR/1, Mux/3
  Delay25/1 -> Switch7/1
  Delay23/1 -> Switch7/3
  Detect Rise Positive/1 -> Switch27/2, Switch1/2, Switch2/2, Switch5/2, OR/3, Subsystem/1(Set), Mux/1, Switch7/2
  Switch7/1 -> Delay23/1, Switch6/1
  last_opt_index/1 -> Delay25/1
  Delay24/1 -> index_voltage/1
  Saturation/1 -> Delay24/1, finite_control_set/4(index)
  trigger_prediction_done/1 -> Delay22/1
  Switch6/1 -> Saturation/1
  [index] -> Switch6/3
  Switch/1 -> [index]
  Subsystem/1(Q) -> Switch6/2  "Q"
  Delay1/1 -> voltages_done/1
  Subsystem/2(!Q) -> Terminator/1
  OR/1 -> Delay1/1, Switch4/2, Switch3/2  "trigger"
  Delay21/1 -> OR/2, Mux/2, Subsystem/2(Reset)
  trigger_delay_comp_done/1 -> Delay21/1
  Delay18/1 -> pu_ux_AXI/1
  Delay20/1 -> pu_ud_AXI/1
  Delay19/1 -> pu_uq_AXI/1
  Delay17/1 -> pu_uy_AXI/1
  Delay15/1 -> Switch5/1
  Switch5/1 -> Delay16/1, Switch/2
  index_select/1 -> Delay15/1
  Delay16/1 -> Switch5/3
  Delay13/1 -> Switch4/1
  Switch4/1 -> Delay14/1, Switch/3
  index_AXI/1 -> Delay13/1
  Delay14/1 -> Switch4/3
  Delay12/1 -> Switch3/1
  Delay11/1 -> Switch2/1
  Delay10/1 -> Switch1/1
  Delay9/1 -> Switch27/1
  Delay8/1 -> Switch3/3
  index/1 -> Delay12/1
  Switch3/1 -> Switch/1, Delay8/1
  Delay7/1 -> pu_ud/1
  Delay6/1 -> pu_uq/1
  Delay5/1 -> pu_ux/1
  Delay4/1 -> pu_uy/1
  Switch2/1 -> Delay3/1, finite_control_set/3(cos_angle)
  Delay3/1 -> Switch2/3
  cos_angle/1 -> Delay11/1
  Switch1/1 -> Delay2/1, finite_control_set/2(sin_angle)
  Delay2/1 -> Switch1/3
  sin_angle/1 -> Delay10/1
  Switch27/1 -> finite_control_set/1(v_DC_pu), Delay56/1
  v_DC_pu/1 -> Delay9/1
  Delay56/1 -> Switch27/3
  Delay/1 -> Detect Rise Positive/1
  trigger_adc/1 -> Delay/1
  finite_control_set/4(pu_uy) -> Delay4/1, Delay17/1
  finite_control_set/3(pu_ux) -> Delay5/1, Delay18/1
  finite_control_set/2(pu_uq) -> Delay6/1, Delay19/1
  finite_control_set/1(pu_ud) -> Delay7/1, Delay20/1

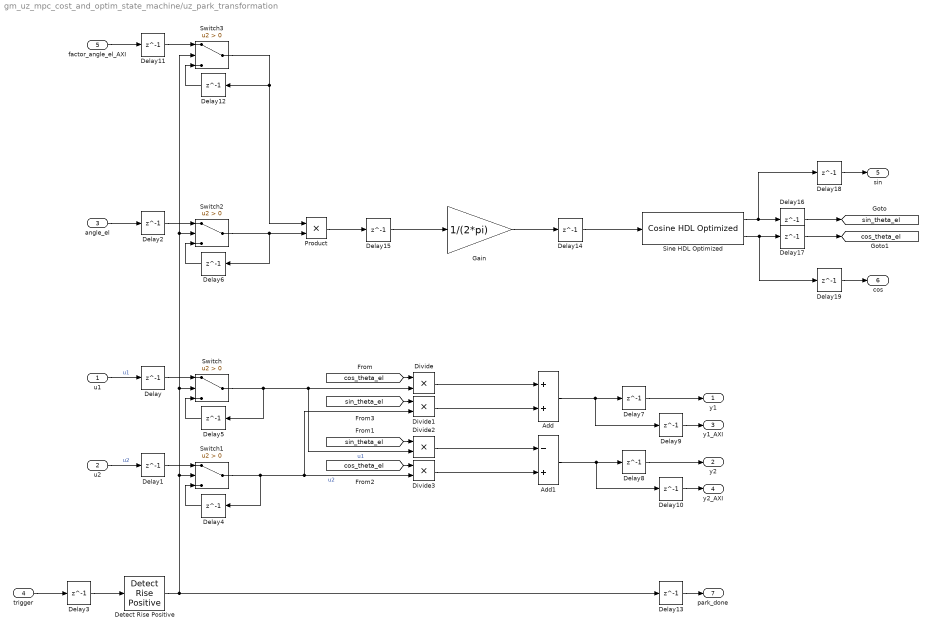
== system gm_uz_mpc_cost_and_optim_state_machine/uz_park_transformation ==
  u1 : Inport
  u2 : Inport  Port=2
  angle_el : Inport  Port=3
  trigger : Inport  Port=4
  factor_angle_el_AXI : Inport  Port=5
  Add : Sum  OutDataTypeStr=fixdt(1,27,16)
  Add1 : Sum  Inputs=-+  OutDataTypeStr=fixdt(1,27,16)
  Delay{,1..19} (20 alike) : Delay  DelayLength=1
  Detect Rise Positive : simulink/Logic and Bit Operations/Detect Rise Positive  vinit=0  OutDataTypeStr=boolean
  Divide{,1..3} (4 alike) : Product  Inputs=**  OutDataTypeStr=fixdt(1,27,16)
  Gain : Gain  Gain=1/(2*pi)  OutDataTypeStr=fixdt(1,18,16)
  Product : Product  OutDataTypeStr=fixdt(1,18,14)
  Sine HDL Optimized : hdlsllib/Lookup Tables/Cosine HDL Optimized  OutputFormula=sin(2*pi*u) and cos(2*pi*u)  NumDataPoints=256  TableDataTypeStr=fixdt(0,17,16)  SimulateLUTROMDelay=off
      settings: SourceProductBaseCode=SL
  Switch{,1..3} (4 alike) : Switch  Criteria=u2 > Threshold
  y1 : Outport  VectorParamsAs1DForOutWhenUnconnected=off
  y2 : Outport  Port=2  VectorParamsAs1DForOutWhenUnconnected=off
  y1_AXI : Outport  Port=3  VectorParamsAs1DForOutWhenUnconnected=off
  y2_AXI : Outport  Port=4  VectorParamsAs1DForOutWhenUnconnected=off
  sin : Outport  Port=5  VectorParamsAs1DForOutWhenUnconnected=off
  cos : Outport  Port=6  VectorParamsAs1DForOutWhenUnconnected=off
  park_done : Outport  Port=7  VectorParamsAs1DForOutWhenUnconnected=off
  tag scope: cos_theta_el=global, sin_theta_el=global
  wires:
  Delay19/1 -> cos/1
  Delay18/1 -> sin/1
  Delay17/1 -> [cos_theta_el]
  Delay16/1 -> [sin_theta_el]
  Delay14/1 -> Sine HDL Optimized/1
  Delay15/1 -> Gain/1
  Delay13/1 -> park_done/1
  Delay3/1 -> Detect Rise Positive/1
  Product/1 -> Delay15/1
  Delay11/1 -> Switch3/1
  Delay12/1 -> Switch3/3
  Detect Rise Positive/1 -> Switch2/2, Switch3/2, Switch/2, Switch1/2, Delay13/1
  factor_angle_el_AXI/1 -> Delay11/1
  Switch3/1 -> Delay12/1, Product/1
  Switch2/1 -> Delay6/1, Product/2
  Delay10/1 -> y2_AXI/1
  Delay9/1 -> y1_AXI/1
  Delay8/1 -> y2/1
  Delay7/1 -> y1/1
  Delay6/1 -> Switch2/3
  Delay5/1 -> Switch/3
  Delay4/1 -> Switch1/3
  trigger/1 -> Delay3/1
  Delay2/1 -> Switch2/1
  Delay1/1 -> Switch1/1
  Delay/1 -> Switch/1
  u2/1 -> Delay1/1  "u2"
  u1/1 -> Delay/1  "u1"
  Gain/1 -> Delay14/1
  Sine HDL Optimized/1 -> Delay16/1, Delay18/1
  Sine HDL Optimized/2 -> Delay17/1, Delay19/1
  angle_el/1 -> Delay2/1
  Divide/1 -> Add/1
  Add1/1 -> Delay8/1, Delay10/1
  Add/1 -> Delay7/1, Delay9/1
  [sin_theta_el] -> Divide1/1
  [cos_theta_el] -> Divide/1
  Divide1/1 -> Add/2
  [sin_theta_el] -> Divide2/1
  Switch/1 -> Delay5/1, Divide/2, Divide2/2  "u1"
  [cos_theta_el] -> Divide3/1
  Divide3/1 -> Add1/2
  Divide2/1 -> Add1/1
  Switch1/1 -> Divide3/2, Divide1/2, Delay4/1  "u2"

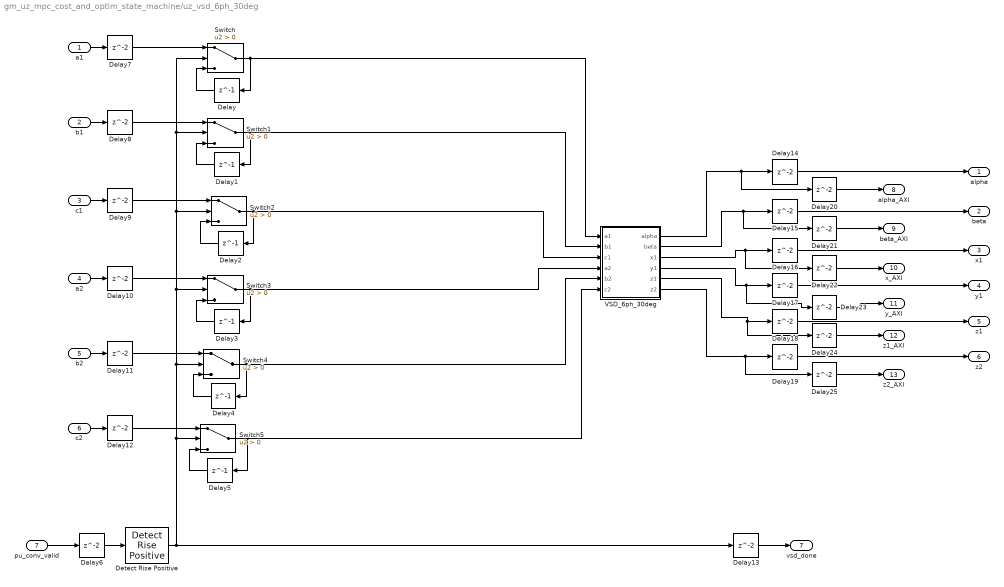
== system gm_uz_mpc_cost_and_optim_state_machine/uz_vsd_6ph_30deg ==
  a1 : Inport
  b1 : Inport  Port=2
  c1 : Inport  Port=3
  a2 : Inport  Port=4
  b2 : Inport  Port=5
  c2 : Inport  Port=6
  pu_conv_valid : Inport  Port=7
  Delay{,1..5} (6 alike) : Delay  DelayLength=1
  Delay{6..25} (20 alike) : Delay
  Detect Rise Positive : simulink/Logic and Bit Operations/Detect Rise Positive  vinit=0  OutDataTypeStr=boolean
  Switch{,1..5} (6 alike) : Switch  Criteria=u2 > Threshold  OutDataTypeStr=fixdt_type_vsd
  VSD_6ph_30deg : MATLAB Function  TreatAsAtomicUnit=on
  alpha : Outport  OutDataTypeStr=fixdt(1,18,11)  VectorParamsAs1DForOutWhenUnconnected=off
  beta : Outport  Port=2  OutDataTypeStr=fixdt(1,18,11)  VectorParamsAs1DForOutWhenUnconnected=off
  x1 : Outport  Port=3  OutDataTypeStr=fixdt(1,18,11)  VectorParamsAs1DForOutWhenUnconnected=off
  y1 : Outport  Port=4  OutDataTypeStr=fixdt(1,18,11)  VectorParamsAs1DForOutWhenUnconnected=off
  z1 : Outport  Port=5  OutDataTypeStr=fixdt(1,18,11)  VectorParamsAs1DForOutWhenUnconnected=off
  z2 : Outport  Port=6  OutDataTypeStr=fixdt(1,18,11)  VectorParamsAs1DForOutWhenUnconnected=off
  vsd_done : Outport  Port=7  VectorParamsAs1DForOutWhenUnconnected=off
  alpha_AXI : Outport  Port=8  OutDataTypeStr=fixdt(1,18,11)  VectorParamsAs1DForOutWhenUnconnected=off
  beta_AXI : Outport  Port=9  OutDataTypeStr=fixdt(1,18,11)  VectorParamsAs1DForOutWhenUnconnected=off
  x_AXI : Outport  Port=10  OutDataTypeStr=fixdt(1,18,11)  VectorParamsAs1DForOutWhenUnconnected=off
  y_AXI : Outport  Port=11  OutDataTypeStr=fixdt(1,18,11)  VectorParamsAs1DForOutWhenUnconnected=off
  z1_AXI : Outport  Port=12  OutDataTypeStr=fixdt(1,18,11)  VectorParamsAs1DForOutWhenUnconnected=off
  z2_AXI : Outport  Port=13  OutDataTypeStr=fixdt(1,18,11)  VectorParamsAs1DForOutWhenUnconnected=off
  wires:
  Delay25/1 -> z2_AXI/1
  Delay24/1 -> z1_AXI/1
  Delay23/1 -> y_AXI/1
  Delay22/1 -> x_AXI/1
  Delay21/1 -> beta_AXI/1
  Delay20/1 -> alpha_AXI/1
  Delay19/1 -> z2/1
  Delay18/1 -> z1/1
  Delay17/1 -> y1/1
  Delay16/1 -> x1/1
  Delay15/1 -> beta/1
  Delay14/1 -> alpha/1
  Delay13/1 -> vsd_done/1
  Delay12/1 -> Switch5/1
  Delay11/1 -> Switch4/1
  Delay10/1 -> Switch3/1
  Delay9/1 -> Switch2/1
  Delay8/1 -> Switch1/1
  Delay7/1 -> Switch/1
  Delay6/1 -> Detect Rise Positive/1
  c2/1 -> Delay12/1
  b2/1 -> Delay11/1
  a2/1 -> Delay10/1
  c1/1 -> Delay9/1
  b1/1 -> Delay8/1
  a1/1 -> Delay7/1
  Switch5/1 -> Delay5/1, VSD_6ph_30deg/6(c2)
  Delay5/1 -> Switch5/3
  Switch4/1 -> Delay4/1, VSD_6ph_30deg/5(b2)
  Delay4/1 -> Switch4/3
  Switch3/1 -> Delay3/1, VSD_6ph_30deg/4(a2)
  Delay3/1 -> Switch3/3
  Switch2/1 -> Delay2/1, VSD_6ph_30deg/3(c1)
  Delay2/1 -> Switch2/3
  Switch1/1 -> Delay1/1, VSD_6ph_30deg/2(b1)
  Delay1/1 -> Switch1/3
  Switch/1 -> Delay/1, VSD_6ph_30deg/1(a1)
  Delay/1 -> Switch/3
  Detect Rise Positive/1 -> Delay13/1, Switch/2, Switch1/2, Switch2/2, Switch3/2, Switch4/2, Switch5/2
  pu_conv_valid/1 -> Delay6/1
  VSD_6ph_30deg/6(z2) -> Delay19/1, Delay25/1
  VSD_6ph_30deg/5(z1) -> Delay18/1, Delay24/1
  VSD_6ph_30deg/4(y1) -> Delay17/1, Delay23/1
  VSD_6ph_30deg/3(x1) -> Delay16/1, Delay22/1
  VSD_6ph_30deg/2(beta) -> Delay15/1, Delay21/1
  VSD_6ph_30deg/1(alpha) -> Delay14/1, Delay20/1

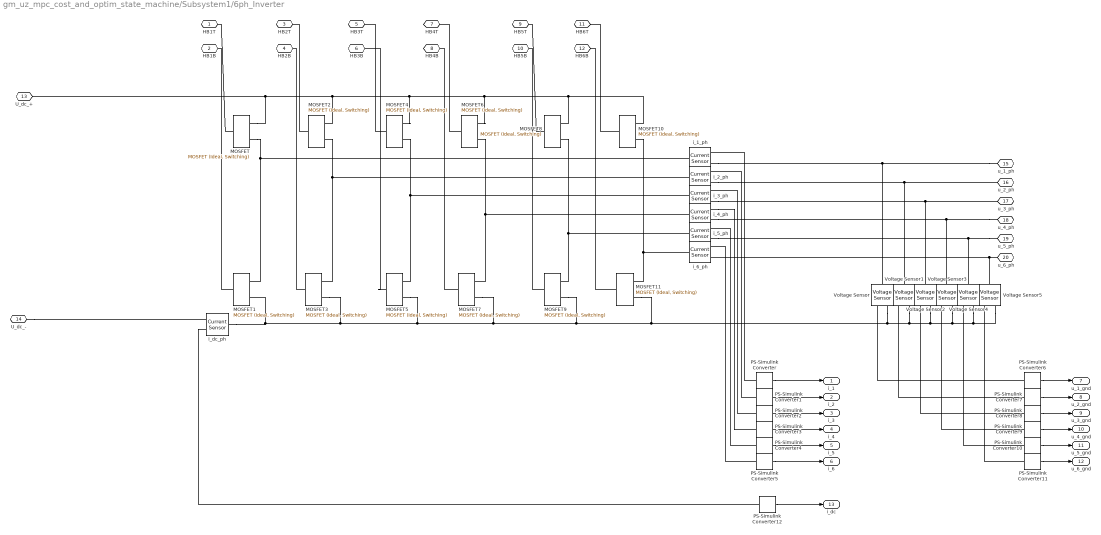
== system gm_uz_mpc_cost_and_optim_state_machine/Subsystem1/6ph_Inverter ==
  MOSFET{,1..11} (12 alike) : ee_lib/Semiconductors & Converters/MOSFET (Ideal, Switching)  Rds=RDSon Ohm  Goff=1e-6 1/Ohm  Vth=0.7 V  diode_param=1  diode_Vf=0.8 V  diode_Ron=0.001 Ohm  diode_Goff=1e-5 1/Ohm  diode_C=5e-8 F  diode_iRM=-235 A  diode_iF=300 A  diode_idot=-50 A/us  diode_trr_param=1  diode_trr_factor=3  diode_trr=15 us  diode_Qrr=1.5e+3 s*uA  thermal_loss_option=ee.enum.converters.thermalLossOption.constantvalues  Von_data=[0, 1.1, 1.3, 1.45, 1.75, 2.25, 2.7; 0, 1, 1.15, 1.35, 1.7, 2.35, 3] V  Eon_data=[0, .29, 1.43, 2.86, 5.71, 13.14, 22.86; 0, .57, 2.63, 5.14, 10.29, 20.57, 30.29] * 1e-3 J  Eoff_data=[0, .21, 1.07, 2.14, 4.29, 9.86, 17.14; 0, .43, 1.97, 3.86, 7.71, 15.43, 22.71] * 1e-3 J  Tj=[298.15, 398.15] K  Iout_data=[0, 10, 50, 100, 200, 400, 600] A  Eon_scalar=22.86e-3 J  Eoff_scalar=17.14e-3 J  Voff=300 V  Iout_scalar=600 A  diodeModelType=ee.enum.converters.diodeModelType.pwl  diode_IfMat=[.07, .12, .19, 1.75, 4.24, 7.32, 11.2; .16, .3, .72, 2.14, 4.02, 6.35, 9.12] A  diode_TjVec=[25, 125] degC  diode_VfVec=[.5, .7, .9, 1.3, 1.7, 2.1, 2.5] V  thermal_network_parameterization=ee.enum.thermalNetworkTopology.external  Rth=[.03, .2] K/W  Rth_Foster=[.03, .2] K/W  thermal_mass_parameterization=ee.enum.thermalNetwork.timeconstant  thermal_mass=[3, 25] J/K  thermal_mass_Foster=[33, 50] J/K  thermal_time_constant=[.1, 5] s  thermal_time_constant_Foster=[1, 10] s  thermal_mass_initial_temperatures=[25, 25] degC  junction_thermal_mass=0.1 J/K  vT_specify=off  vT_priority=None  vT=0 V  vT_nominal_specify=off  vT_nominal_unit=V  vT_nominal_value=1  Qj_specify=off  Qj_priority=None  Qj=0 W  Qj_nominal_specify=off  Qj_nominal_unit=W  Qj_nominal_value=1  junction_temperature_specify=off  junction_temperature_priority=None  junction_temperature=25 degC  junction_temperature_nominal_specify=off  junction_temperature_nominal_unit=degC  junction_temperature_nominal_value=1
  PS-Simulink Converter{,1..5,12} (7 alike) : nesl_utility/PS-Simulink Converter  PhysicalDomain=network_engine_domain  SubClassName=ps_output  LeftPortType=input  RightPortType=output  PseudoPeriodic=off  Frequencies=[]  Unit=A  AffineConversion=off
  PS-Simulink Converter{6..11} (6 alike) : nesl_utility/PS-Simulink Converter  PhysicalDomain=network_engine_domain  SubClassName=ps_output  LeftPortType=input  RightPortType=output  PseudoPeriodic=off  Frequencies=[]  Unit=V  AffineConversion=off
  Voltage Sensor{,1..5} (6 alike) : fl_lib/Electrical/Electrical Sensors/Voltage Sensor
  i_1_ph : fl_lib/Electrical/Electrical Sensors/Current Sensor
  i_2_ph : fl_lib/Electrical/Electrical Sensors/Current Sensor
  i_3_ph : fl_lib/Electrical/Electrical Sensors/Current Sensor
  i_4_ph : fl_lib/Electrical/Electrical Sensors/Current Sensor
  i_5_ph : fl_lib/Electrical/Electrical Sensors/Current Sensor
  i_6_ph : fl_lib/Electrical/Electrical Sensors/Current Sensor
  i_dc_ph : fl_lib/Electrical/Electrical Sensors/Current Sensor
  HB1T : PMIOPort  Side=Left
  HB1B : PMIOPort  Port=2  Side=Left
  HB2T : PMIOPort  Port=3  Side=Left
  HB2B : PMIOPort  Port=4  Side=Left
  HB3T : PMIOPort  Port=5  Side=Left
  HB3B : PMIOPort  Port=6  Side=Left
  HB4T : PMIOPort  Port=7  Side=Left
  HB4B : PMIOPort  Port=8  Side=Left
  HB5T : PMIOPort  Port=9  Side=Left
  HB5B : PMIOPort  Port=10  Side=Left
  HB6T : PMIOPort  Port=11  Side=Left
  HB6B : PMIOPort  Port=12  Side=Left
  U_dc_+ : PMIOPort  Port=13  Side=Left
  U_dc_- : PMIOPort  Port=14  Side=Left
  u_1_ph : PMIOPort  Port=15  Side=Right
  u_2_ph : PMIOPort  Port=16  Side=Right
  u_3_ph : PMIOPort  Port=17  Side=Right
  u_4_ph : PMIOPort  Port=18  Side=Right
  u_5_ph : PMIOPort  Port=19  Side=Right
  u_6_ph : PMIOPort  Port=20  Side=Right
  i_1 : Outport  VectorParamsAs1DForOutWhenUnconnected=off
  i_2 : Outport  Port=2  VectorParamsAs1DForOutWhenUnconnected=off
  i_3 : Outport  Port=3  VectorParamsAs1DForOutWhenUnconnected=off
  i_4 : Outport  Port=4  VectorParamsAs1DForOutWhenUnconnected=off
  i_5 : Outport  Port=5  VectorParamsAs1DForOutWhenUnconnected=off
  i_6 : Outport  Port=6  VectorParamsAs1DForOutWhenUnconnected=off
  u_1_gnd : Outport  Port=7  VectorParamsAs1DForOutWhenUnconnected=off
  u_2_gnd : Outport  Port=8  VectorParamsAs1DForOutWhenUnconnected=off
  u_3_gnd : Outport  Port=9  VectorParamsAs1DForOutWhenUnconnected=off
  u_4_gnd : Outport  Port=10  VectorParamsAs1DForOutWhenUnconnected=off
  u_5_gnd : Outport  Port=11  VectorParamsAs1DForOutWhenUnconnected=off
  u_6_gnd : Outport  Port=12  VectorParamsAs1DForOutWhenUnconnected=off
  i_dc : Outport  Port=13  VectorParamsAs1DForOutWhenUnconnected=off
  wires:
  PS-Simulink Converter12/1 -> i_dc/1
  PS-Simulink Converter11/1 -> u_6_gnd/1
  PS-Simulink Converter10/1 -> u_5_gnd/1
  PS-Simulink Converter6/1 -> u_1_gnd/1
  PS-Simulink Converter7/1 -> u_2_gnd/1
  PS-Simulink Converter8/1 -> u_3_gnd/1
  PS-Simulink Converter9/1 -> u_4_gnd/1
  PS-Simulink Converter5/1 -> i_6/1
  PS-Simulink Converter4/1 -> i_5/1
  PS-Simulink Converter3/1 -> i_4/1
  PS-Simulink Converter2/1 -> i_3/1
  PS-Simulink Converter1/1 -> i_2/1
  PS-Simulink Converter/1 -> i_1/1
  connections:
  MOSFET8/RConn1 -- MOSFET10/RConn1 -- MOSFET4/RConn1 -- MOSFET2/RConn1 -- U_dc_+/RConn1 -- MOSFET/RConn1 -- MOSFET6/RConn1
  PS-Simulink Converter12/LConn1 -- i_dc_ph/RConn1
  U_dc_-/RConn1 -- i_dc_ph/RConn2
  PS-Simulink Converter11/LConn1 -- Voltage Sensor5/RConn1
  PS-Simulink Converter10/LConn1 -- Voltage Sensor4/RConn1
  PS-Simulink Converter9/LConn1 -- Voltage Sensor3/RConn1
  PS-Simulink Converter8/LConn1 -- Voltage Sensor2/RConn1
  PS-Simulink Converter7/LConn1 -- Voltage Sensor1/RConn1
  PS-Simulink Converter6/LConn1 -- Voltage Sensor/RConn1
  PS-Simulink Converter5/LConn1 -- i_6_ph/RConn1
  PS-Simulink Converter4/LConn1 -- i_5_ph/RConn1
  i_4_ph/RConn1 -- PS-Simulink Converter3/LConn1
  PS-Simulink Converter2/LConn1 -- i_3_ph/RConn1
  PS-Simulink Converter1/LConn1 -- i_2_ph/RConn1
  PS-Simulink Converter/LConn1 -- i_1_ph/RConn1
  Voltage Sensor5/LConn1 -- i_6_ph/RConn2 -- u_6_ph/RConn1
  u_5_ph/RConn1 -- Voltage Sensor4/LConn1 -- i_5_ph/RConn2
  u_4_ph/RConn1 -- Voltage Sensor3/LConn1 -- i_4_ph/RConn2
  Voltage Sensor2/LConn1 -- u_3_ph/RConn1 -- i_3_ph/RConn2
  Voltage Sensor1/LConn1 -- u_2_ph/RConn1 -- i_2_ph/RConn2
  u_1_ph/RConn1 -- Voltage Sensor/LConn1 -- i_1_ph/RConn2
  MOSFET3/LConn1 -- HB2B/RConn1
  MOSFET6/LConn1 -- HB4T/RConn1
  MOSFET10/LConn1 -- HB6T/RConn1
  MOSFET4/LConn1 -- HB3T/RConn1
  MOSFET8/LConn1 -- HB5T/RConn1
  MOSFET7/LConn1 -- HB4B/RConn1
  MOSFET1/LConn1 -- HB1B/RConn1
  MOSFET5/LConn1 -- HB3B/RConn1
  MOSFET9/LConn1 -- HB5B/RConn1
  MOSFET/LConn1 -- HB1T/RConn1
  MOSFET11/RConn1 -- i_6_ph/LConn1 -- MOSFET10/RConn2
  MOSFET2/LConn1 -- HB2T/RConn1
  MOSFET9/RConn1 -- i_5_ph/LConn1 -- MOSFET8/RConn2
  MOSFET11/LConn1 -- HB6B/RConn1
  MOSFET1/RConn1 -- i_1_ph/LConn1 -- MOSFET/RConn2
  MOSFET3/RConn2 -- MOSFET1/RConn2 -- i_dc_ph/LConn1 -- MOSFET7/RConn2 -- MOSFET9/RConn2 -- MOSFET11/RConn2 -- Voltage Sensor/RConn2 -- Voltage Sensor1/RConn2 -- Voltage Sensor2/RConn2 -- Voltage Sensor3/RConn2 -- Voltage Sensor4/RConn2 -- Voltage Sensor5/RConn2 -- MOSFET5/RConn2
  MOSFET5/RConn1 -- i_3_ph/LConn1 -- MOSFET4/RConn2
  MOSFET3/RConn1 -- i_2_ph/LConn1 -- MOSFET2/RConn2
  MOSFET7/RConn1 -- i_4_ph/LConn1 -- MOSFET6/RConn2

== system gm_uz_mpc_cost_and_optim_state_machine/Subsystem1/DC_link ==
  Capacitor : fl_lib/Electrical/Electrical Elements/Capacitor  c=C_dc_link uF  r=1e-6 Ohm  g=0 1/Ohm  i_specify=off  i_priority=None  i=0 A  i_nominal_specify=off  i_nominal_unit=A  i_nominal_value=1  v_specify=off  v_priority=None  v=0 V  v_nominal_specify=off  v_nominal_unit=V  v_nominal_value=1  vc_specify=off  vc_priority=High  vc=0 V  vc_nominal_specify=off  vc_nominal_unit=V  vc_nominal_value=1
  PS-Simulink Converter : nesl_utility/PS-Simulink Converter  PhysicalDomain=network_engine_domain  SubClassName=ps_output  LeftPortType=input  RightPortType=output  PseudoPeriodic=off  Frequencies=[]  Unit=1  AffineConversion=off
      settings: SourceProductBaseCode=PW,SS
  Voltage Sensor : fl_lib/Electrical/Electrical Sensors/Voltage Sensor
  U_dc_link+_in : PMIOPort  Side=Left
  U_dc_link-_in : PMIOPort  Port=2  Side=Left
  U_dc_link+_out : PMIOPort  Port=3  Side=Right
  U_dc_link-_out : PMIOPort  Port=4  Side=Right
  u_dc_link_measured : Outport  VectorParamsAs1DForOutWhenUnconnected=off
  wires:
  PS-Simulink Converter/1 -> u_dc_link_measured/1
  connections:
  Voltage Sensor/RConn1 -- PS-Simulink Converter/LConn1
  Capacitor/RConn1 -- U_dc_link-_out/RConn1 -- Voltage Sensor/RConn2 -- U_dc_link-_in/RConn1
  Capacitor/LConn1 -- U_dc_link+_out/RConn1 -- Voltage Sensor/LConn1 -- U_dc_link+_in/RConn1

== system gm_uz_mpc_cost_and_optim_state_machine/Subsystem1/Power_Source ==
  Controlled Voltage Source : fl_lib/Electrical/Electrical Sources/Controlled Voltage Source
  + : PMIOPort  Side=Right
  - : PMIOPort  Port=2  Side=Right
  ref_voltage : PMIOPort  Port=3  Side=Left
  connections:
  Controlled Voltage Source/RConn1 -- ref_voltage/RConn1
  Controlled Voltage Source/RConn2 -- -/RConn1
  Controlled Voltage Source/LConn1 -- +/RConn1
